simulink model "quad_model"  (R2025b)
settings: Solver=VariableStepAuto  StartTime=0.0  StopTime=10.0  RelTol=1e-3
values from neighbouring files (symbols this model uses):
  Cd = diag([0.10 0.10 0.15])    [quad_params.m]
  g = 9.81    [quad_params.m]
  h0 = 2    [quad_params.m]
  Ivec = [Ixx; Iyy; Izz]    [quad_params.m]
  m = 1.20    (= 1.2)    [quad_params.m]
  MIX = [ kT     kT     kT     kT ... (first row only)    [quad_params.m]
  om0 = [0; 0; 0]    [quad_params.m]
  tau = 0.05    [quad_params.m]
  w_max = 1200    [quad_params.m]
settings Model: Creator=chris  LastModifiedBy=chris
settings ModelReferenceCC: ModelReferenceMinAlgLoopOccurrences=on

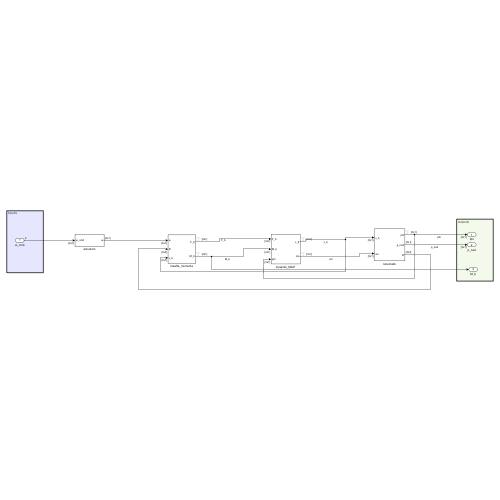
[thumbnail: Simulink's stored preview of the top-level diagram]
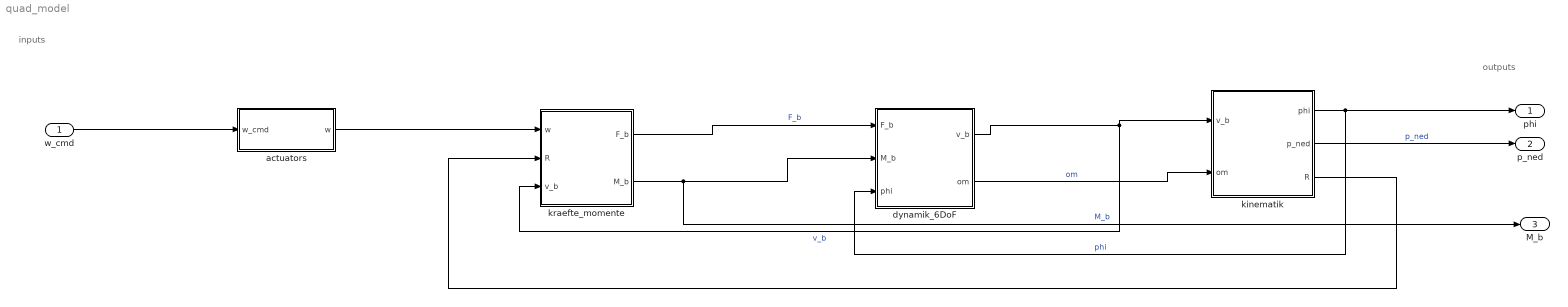
== system quad_model ==
  note: inputs
  note: outputs
  w_cmd : Inport  PortDimensions=4
  actuators : Subsystem
  dynamik_6DoF : Subsystem
  kinematik : Subsystem
  kraefte_momente : Subsystem
  phi : Outport  PortDimensions=[3 1]
  p_ned : Outport  Port=2
  M_b : Outport  Port=3
  wires:
  actuators/1(w) -> kraefte_momente/1(w)
  kraefte_momente/1(F_b) -> dynamik_6DoF/1(F_b)  "F_b"
  kraefte_momente/2(M_b) -> M_b/1, dynamik_6DoF/2(M_b)  "M_b"
  dynamik_6DoF/1(v_b) -> kinematik/1(v_b), kraefte_momente/3(v_b)  "v_b"
  dynamik_6DoF/2(om) -> kinematik/2(om)  "om"
  kinematik/3(R) -> kraefte_momente/2(R)
  kinematik/1(phi) -> dynamik_6DoF/3(phi), phi/1  "phi"
  kinematik/2(p_ned) -> p_ned/1  "p_ned"
  w_cmd/1 -> actuators/1(w_cmd)

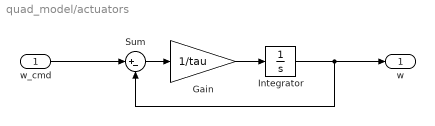
== system quad_model/actuators ==
  w_cmd : Inport  PortDimensions=[4 1]
  Gain : Gain  Gain=1/tau
  Integrator : Integrator  InitialCondition=zeros(4,1)  LimitOutput=on  UpperSaturationLimit=w_max  LowerSaturationLimit=0  IgnoreLimit=on
  Sum : Sum  Inputs=|+-
  w : Outport  PortDimensions=[4 1]
  wires:
  Sum/1 -> Gain/1
  Gain/1 -> Integrator/1
  w_cmd/1 -> Sum/1
  Integrator/1 -> Sum/2, w/1

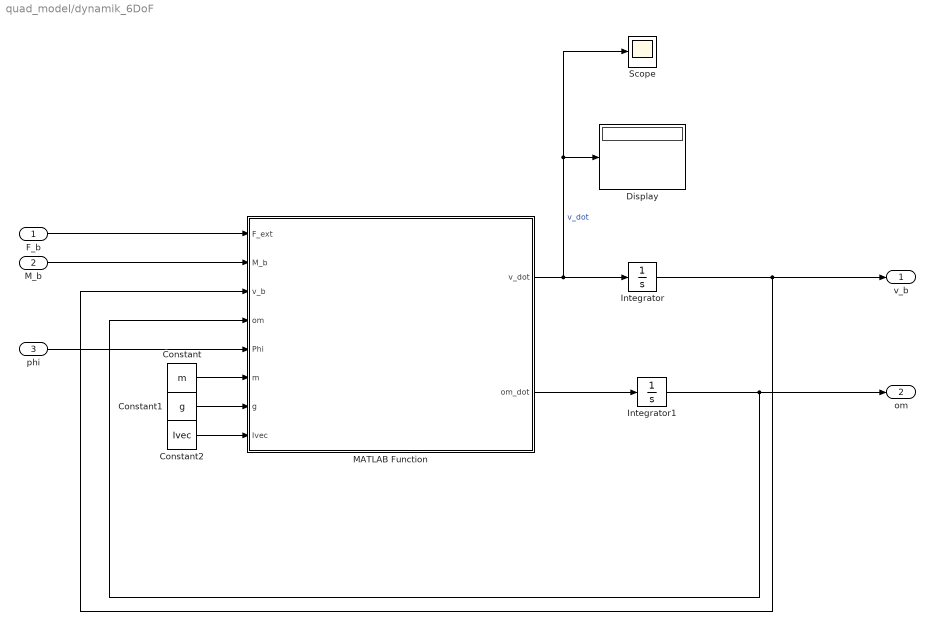
== system quad_model/dynamik_6DoF ==
  F_b : Inport  PortDimensions=[3 1]
  M_b : Inport  Port=2  PortDimensions=[3 1]
  phi : Inport  Port=3  PortDimensions=[3 1]
  Constant : Constant  Value=m
  Constant1 : Constant  Value=g
  Constant2 : Constant  Value=Ivec
  Display : Display
  Integrator : Integrator  InitialCondition=[0;0;0]
  Integrator1 : Integrator  InitialCondition=om0
  MATLAB Function : MATLAB Function  TreatAsAtomicUnit=on
  Scope : Scope
      settings: ActiveDisplayYMinimum=-3.3891115314769991  ActiveDisplayYMaximum=23.649700968523
  v_b : Outport  PortDimensions=[3 1]
  om : Outport  Port=2  PortDimensions=[3 1]
  wires:
  MATLAB Function/1(v_dot) -> Scope/1, Display/1, Integrator/1  "v_dot"
  MATLAB Function/2(om_dot) -> Integrator1/1
  Constant1/1 -> MATLAB Function/7(g)
  F_b/1 -> MATLAB Function/1(F_ext)
  M_b/1 -> MATLAB Function/2(M_b)
  Constant/1 -> MATLAB Function/6(m)
  Integrator1/1 -> om/1, MATLAB Function/4(om)
  Constant2/1 -> MATLAB Function/8(Ivec)
  Integrator/1 -> v_b/1, MATLAB Function/3(v_b)
  phi/1 -> MATLAB Function/5(Phi)

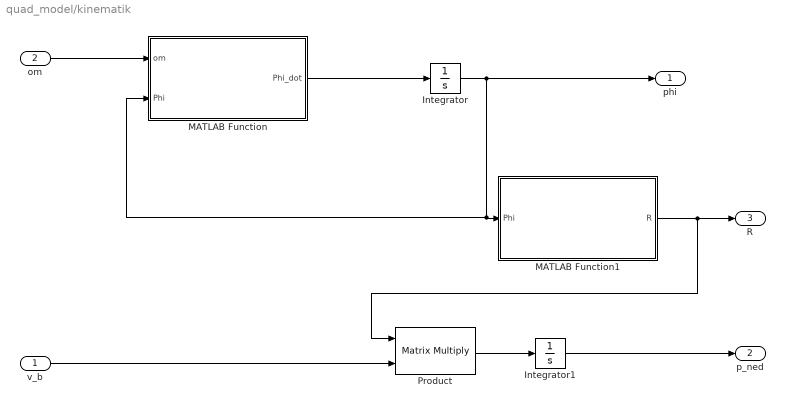
== system quad_model/kinematik ==
  v_b : Inport  PortDimensions=[3 1]
  om : Inport  Port=2  PortDimensions=[3 1]
  Integrator : Integrator  InitialCondition=[0;0;0]
  Integrator1 : Integrator  InitialCondition=[0;0;h0]
  MATLAB Function : MATLAB Function  TreatAsAtomicUnit=on
  MATLAB Function1 : MATLAB Function  TreatAsAtomicUnit=on
  Product : Product  Multiplication=Matrix(*)
  phi : Outport  PortDimensions=[3 1]
  p_ned : Outport  Port=2
  R : Outport  Port=3  PortDimensions=[3 3]
  wires:
  Integrator/1 -> phi/1, MATLAB Function/2(Phi), MATLAB Function1/1(Phi)
  Integrator1/1 -> p_ned/1
  v_b/1 -> Product/2
  MATLAB Function1/1(R) -> Product/1, R/1
  MATLAB Function/1(Phi_dot) -> Integrator/1
  om/1 -> MATLAB Function/1(om)
  Product/1 -> Integrator1/1

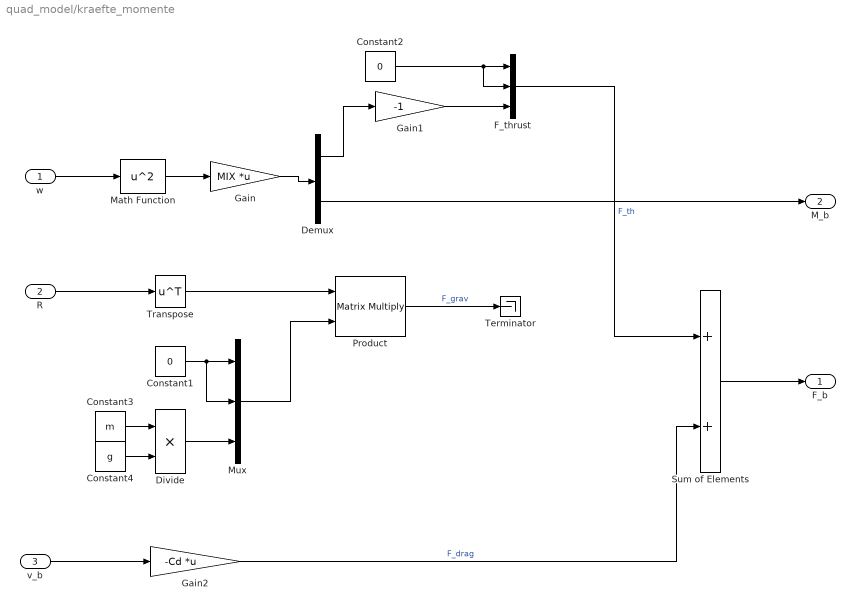
== system quad_model/kraefte_momente ==
  w : Inport  PortDimensions=[4 1]
  R : Inport  Port=2  PortDimensions=[3 3]
  v_b : Inport  Port=3  PortDimensions=[3 1]
  Constant1 : Constant  Value=0
  Constant2 : Constant  Value=0
  Constant3 : Constant  Value=m
  Constant4 : Constant  Value=g
  Demux : Demux  Outputs=[1 3]
  Divide : Product  Inputs=**
  F_thrust : Concatenate  NumInputs=3
  Gain : Gain  Gain=MIX  Multiplication=Matrix(K*u)
  Gain1 : Gain  Gain=-1
  Gain2 : Gain  Gain=-Cd  Multiplication=Matrix(K*u)
  Math Function : Math  Operator=square
  Mux : Mux  Inputs=3
  Product : Product  Multiplication=Matrix(*)
  Sum of Elements : Sum
  Terminator : Terminator
  Transpose : Math  Operator=transpose
  F_b : Outport  PortDimensions=[3 1]
  M_b : Outport  Port=2  PortDimensions=[3 1]
  wires:
  v_b/1 -> Gain2/1
  Constant1/1 -> Mux/2, Mux/1
  Demux/2 -> M_b/1
  Constant4/1 -> Divide/2
  Divide/1 -> Mux/3
  Constant2/1 -> F_thrust/2, F_thrust/1
  w/1 -> Math Function/1
  Constant3/1 -> Divide/1
  Gain2/1 -> Sum of Elements/2  "F_drag"
  Sum of Elements/1 -> F_b/1
  Math Function/1 -> Gain/1
  Mux/1 -> Product/2
  Transpose/1 -> Product/1
  F_thrust/1 -> Sum of Elements/1  "F_th"
  Gain1/1 -> F_thrust/3
  R/1 -> Transpose/1
  Product/1 -> Terminator/1  "F_grav"
  Gain/1 -> Demux/1
  Demux/1 -> Gain1/1

== matlab function quad_model/kinematik/MATLAB Function ==
  data: om input; Phi_dot output; Phi input
function Phi_dot = eulerRates(om, Phi)
phi = Phi(1); the = Phi(2);
sph=sin(phi); cph=cos(phi); cth=cos(the); tth=tan(the);
W = [1, sph*tth, cph*tth;
     0, cph,    -sph;
     0, sph/cth, cph/cth];   % Singularität bei the = ±pi/2
Phi_dot = W * om;
end

== matlab function quad_model/dynamik_6DoF/MATLAB Function ==
  data: F_ext input; v_dot output; M_b input; v_b input; om input; Phi input; m input; g input; Ivec input; om_dot output
function [v_dot, om_dot] = eom_rhs(F_ext, M_b, v_b, om, Phi, m, g, Ivec)
% ... R weiterhin intern berechnen (für die Gravitation!) ...
phi=Phi(1); the=Phi(2); psi=Phi(3);
cph=cos(phi); sph=sin(phi); cth=cos(the); sth=sin(the); cps=cos(psi); sps=sin(psi);
R = [cth*cps, sph*sth*cps-cph*sps, cph*sth*cps+sph*sps;
     cth*sps, sph*sth*sps+cph*cps, cph*sth*sps-sph*cps;
    -sth,     sph*cth,             cph*cth];
F_grav_b = R.' * [0; 0; m*g];
v_dot  = (F_ext + F_grav_b)/m - cross(om, v_b);   % (4.1)
om_dot = (M_b - cross(om, Ivec.*om)) ./ Ivec;     % (4.2)
end

== matlab function quad_model/kinematik/MATLAB Function1 ==
  data: R output; Phi input
function R = buildR(Phi)
phi=Phi(1); the=Phi(2); psi=Phi(3);
cph=cos(phi); sph=sin(phi); cth=cos(the); sth=sin(the); cps=cos(psi); sps=sin(psi);
R = [cth*cps, sph*sth*cps-cph*sps, cph*sth*cps+sph*sps;
     cth*sps, sph*sth*sps+cph*cps, cph*sth*sps-sph*cps;
    -sth,     sph*cth,             cph*cth];
end
